simulink model "RealModel"  (R2016a)
settings: Solver=VariableStepAuto  StartTime=0.0  StopTime=10.0  RelTol=1e-3
undefined symbols (not defined in the file or in its folder): K
(part 2 of 7)

== matlab function RealModel/Modell der Strecke/MATLAB Function ==
  data: x input; x_dot input; T input; x_dotdot_out output
function x_dotdot_out = fcn(x, x_dot, T)

%Zuweisung Koordinaten und Ableitungen
x1 = x(1); %theta_x
x2 = x_dot(1); %theta_y
x3 = x(2);
x4 = x_dot(2);
x5 = x(3);
x6 = x_dot(3);
x7 = x(4);
x8 = x_dot(4);
x9 = x(5);
x10 = x_dot(5);

u1 = T(1);
u2 = T(2);
u3 = T(3);


